simulink model "Buck_Converter_Block_Diagram"  (R2024b)
settings: Solver=VariableStepAuto  StartTime=0.0  StopTime=10.0  RelTol=1e-3
settings Model: Creator=User  LastModifiedBy=User

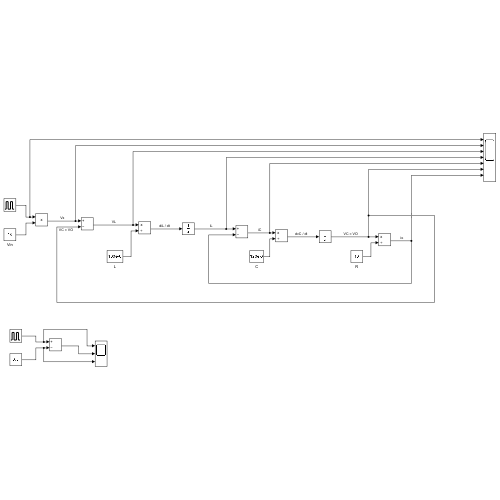
[thumbnail: Simulink's stored preview of the top-level diagram]
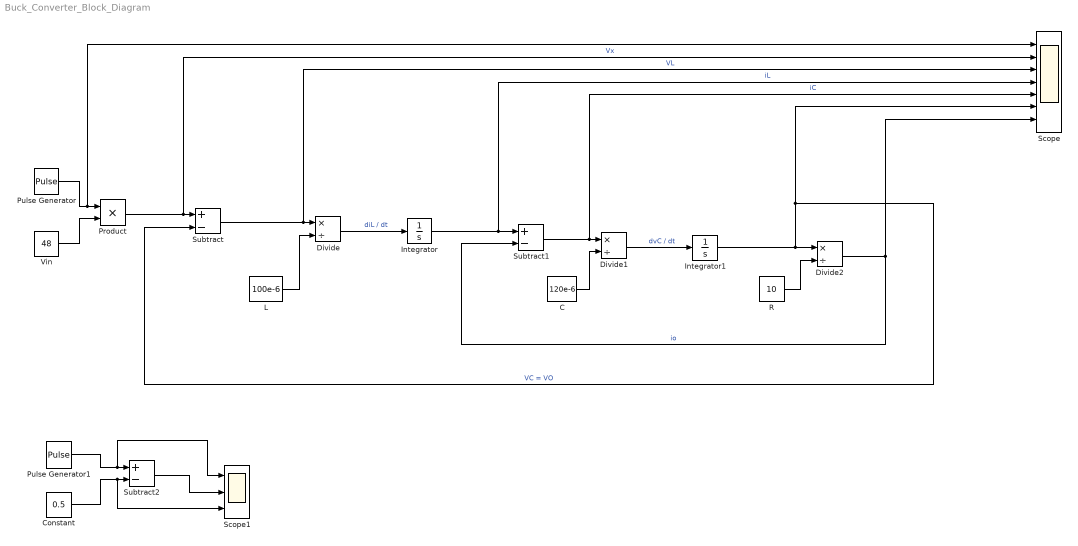
== system Buck_Converter_Block_Diagram ==
  C : Constant  Value=120e-6
  Constant : Constant  Value=0.5
  Divide : Product  Inputs=*/
  Divide1 : Product  Inputs=*/
  Divide2 : Product  Inputs=*/
  Integrator : Integrator
  Integrator1 : Integrator
  L : Constant  Value=100e-6
  Product : Product
  Pulse Generator : DiscretePulseGenerator  PulseType=Time based  Period=1/100e3  PulseWidth=50
  Pulse Generator1 : DiscretePulseGenerator  PulseType=Time based  Period=1/100e3  PulseWidth=50
  R : Constant  Value=10
  Scope : Scope  NumInputPorts=7
  Scope1 : Scope  NumInputPorts=3
  Subtract : Sum  Inputs=+-
  Subtract1 : Sum  Inputs=+-
  Subtract2 : Sum  Inputs=+-
  Vin : Constant  Value=48
  wires:
  Pulse Generator/1 -> Scope/1, Product/1
  Vin/1 -> Product/2
  Product/1 -> Subtract/1, Scope/2  "Vx"
  Subtract/1 -> Scope/3, Divide/1  "VL"
  L/1 -> Divide/2
  Divide/1 -> Integrator/1  "diL / dt"
  Integrator/1 -> Scope/4, Subtract1/1  "iL"
  Subtract1/1 -> Scope/5, Divide1/1  "iC"
  C/1 -> Divide1/2
  Divide1/1 -> Integrator1/1  "dvC / dt"
  Integrator1/1 -> Subtract/2, Scope/6, Divide2/1  "VC = VO"
  R/1 -> Divide2/2
  Divide2/1 -> Scope/7, Subtract1/2  "io"
  Pulse Generator1/1 -> Scope1/1, Subtract2/1
  Constant/1 -> Scope1/3, Subtract2/2
  Subtract2/1 -> Scope1/2
